simulink model "WiperMotor"  (R2025b)
settings: Solver=FixedStepDiscrete  StartTime=0.0  StopTime=20  RelTol=1e-3  EnableMultiTasking=on
settings Model: Creator=Ahmed  LastModifiedBy=Ahmed
settings DataIOCC: SaveOutput=off  SaveTime=off
settings OptimizationCC: DefaultParameterBehavior=Inlined  UseDivisionForNetSlopeComputation=on  GainParamInheritBuiltInType=on  UseFloatMulNetSlope=on  InlineInvariantSignals=on  PassReuseOutputArgsAs=Individual arguments  ZeroExternalMemoryAtStartup=off  ZeroInternalMemoryAtStartup=off  NoFixptDivByZeroProtection=on  EfficientFloat2IntCast=on  LifeSpan=1  OptimizeBlockOrder=speed  DifferentSizesBufferReuse=on  EfficientTunableParamExpr=on
settings DebuggingCC: ParameterTunabilityLossMsg=error
settings HardwareCC: ProdLongLongMode=on
settings ModelReferenceCC: ModelReferenceNumInstancesAllowed=Single
settings SFSimCC: MATLABDynamicMemAlloc=off
settings RTWCC: SystemTargetFile=ert.tlc  GenCodeOnly=on  TemplateMakefile=ert_default_tmf  GenerateReport=on  Description=Embedded Coder
settings CodeAppCC: ForceParamTrailComments=on  IgnoreCustomStorageClasses=off  OperatorAnnotations=on  SimulinkDataObjDesc=on  SFDataObjDesc=on  CustomSymbolStrGlobalVar=rt$N$M  CustomSymbolStrType=$N$M  CustomSymbolStrFcn=$N$M$F  CustomSymbolStrMacro=$N$M  InsertBlockDesc=on
settings ERTTargetCC: ERTCustomFileTemplate=example_file_process.tlc  ERTFilePackagingFormat=CompactWithDataFile  TargetLangStandard=C99 (ISO)  GenerateSampleERTMain=on  IncludeMdlTerminateFcn=off  CombineSignalStateStructs=on  SubcomponentCodeInterfacePackaging=Nonreusable function  SupportComplex=off

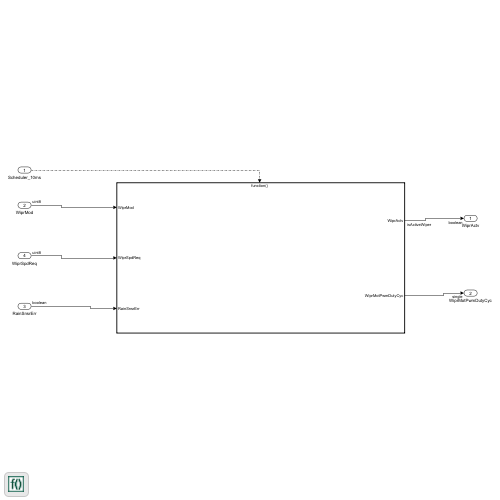
[thumbnail: Simulink's stored preview of the top-level diagram]
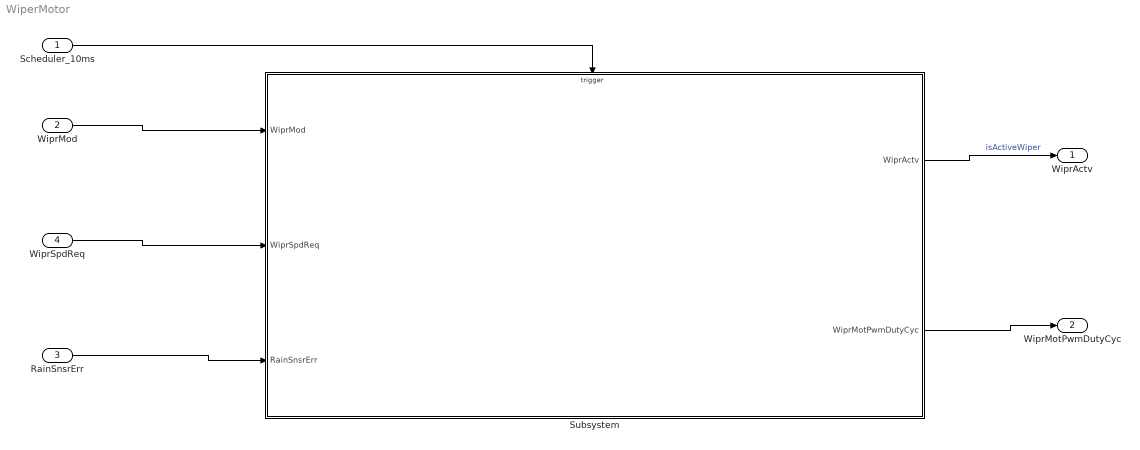
== system WiperMotor ==
  Scheduler_10ms : Inport  PortDimensions=1  OutputFunctionCall=on
  WiprMod : Inport  Port=2  OutDataTypeStr=uint8  PortDimensions=1
  RainSnsrErr : Inport  Port=3  OutDataTypeStr=boolean  PortDimensions=1
  WiprSpdReq : Inport  Port=4  OutDataTypeStr=uint8  PortDimensions=1
  Subsystem : Subsystem
  WiprActv : Outport  OutDataTypeStr=boolean  PortDimensions=1
  WiprMotPwmDutyCyc : Outport  Port=2  OutDataTypeStr=single  PortDimensions=1
  wires:
  WiprMod/1 -> Subsystem/1(WiprMod)
  WiprSpdReq/1 -> Subsystem/2(WiprSpdReq)
  RainSnsrErr/1 -> Subsystem/3(RainSnsrErr)
  Subsystem/1(WiprActv) -> WiprActv/1  "isActiveWiper"
  Subsystem/2(WiprMotPwmDutyCyc) -> WiprMotPwmDutyCyc/1
  Scheduler_10ms/1 -> Subsystem/Trigger

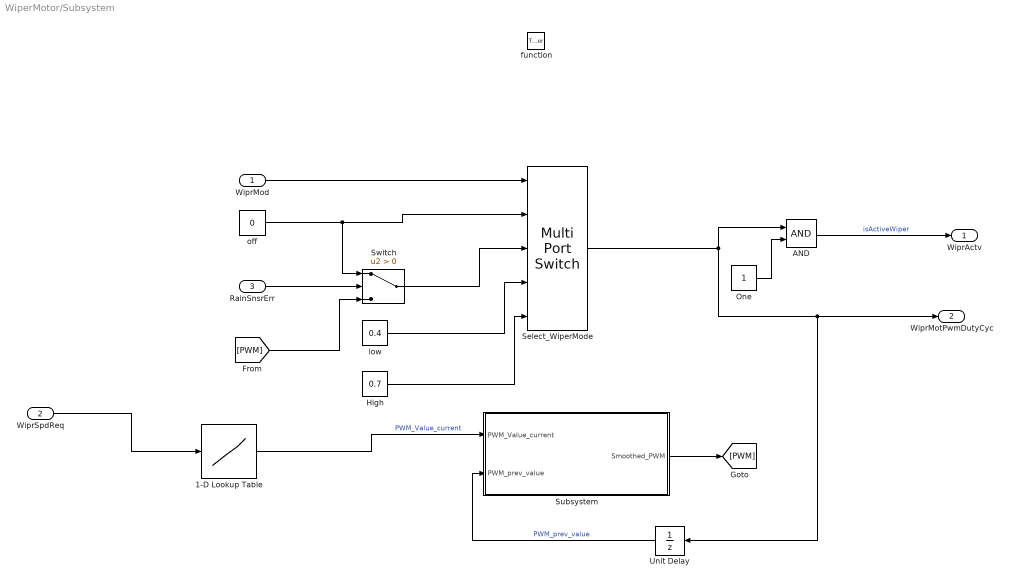
== system WiperMotor/Subsystem ==
  WiprMod : Inport
  WiprSpdReq : Inport  Port=2
  RainSnsrErr : Inport  Port=3
  function : TriggerPort  TriggerType=function-call  VariantControl=(inherit)
  1-D Lookup Table : Lookup_n-D  NumberOfTableDimensions=1  BreakpointsForDimension1=[0,1,2,3,4,5,6,7]  BreakpointsForDimension1DataTypeStr=single  Table=[0, 0.4, 0.45, 0.5, 0.55, 0.6, 0.65, 0.7]  TableDataTypeStr=single  ExtrapMethod=Clip  InternalRulePriority=Speed  OutDataTypeStr=single  RndMeth=Simplest
  AND : Logic  AllPortsSameDT=off  OutDataTypeStr=boolean
  High : Constant  Value=0.7  OutDataTypeStr=Inherit: Inherit via back propagation
  One : Constant  OutDataTypeStr=Inherit: Inherit via back propagation
  Select_WiperMode : MultiPortSwitch  DataPortOrder=Zero-based contiguous  Inputs=4  zeroidx=on  SaturateOnIntegerOverflow=off  InputSameDT=off
  Subsystem : Subsystem
  Switch : Switch  Criteria=u2 > Threshold  SaturateOnIntegerOverflow=off  InputSameDT=off
  Unit Delay : UnitDelay  SampleTime=-1  HasFrameUpgradeWarning=on
  low : Constant  Value=0.4  OutDataTypeStr=Inherit: Inherit via back propagation
  off : Constant  Value=0  OutDataTypeStr=Inherit: Inherit via back propagation
  WiprActv : Outport
  WiprMotPwmDutyCyc : Outport  Port=2
  wires:
  1-D Lookup Table/1 -> Subsystem/1(PWM_Value_current)  "PWM_Value_current"
  WiprSpdReq/1 -> 1-D Lookup Table/1
  [PWM] -> Switch/3
  Subsystem/1(Smoothed_PWM) -> [PWM]
  Unit Delay/1 -> Subsystem/2(PWM_prev_value)  "PWM_prev_value"
  AND/1 -> WiprActv/1  "isActiveWiper"
  One/1 -> AND/2
  Select_WiperMode/1 -> AND/1, WiprMotPwmDutyCyc/1, Unit Delay/1
  High/1 -> Select_WiperMode/5
  low/1 -> Select_WiperMode/4
  RainSnsrErr/1 -> Switch/2
  Switch/1 -> Select_WiperMode/3
  off/1 -> Select_WiperMode/2, Switch/1
  WiprMod/1 -> Select_WiperMode/1

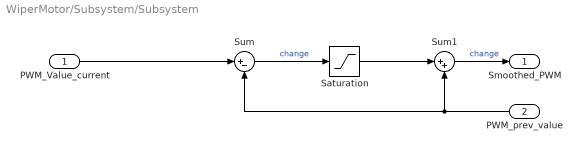
== system WiperMotor/Subsystem/Subsystem ==
  PWM_Value_current : Inport
  PWM_prev_value : Inport  Port=2
  Saturation : Saturate  UpperLimit=0.005  LowerLimit=-0.005
  Sum : Sum  Inputs=|+-
  Sum1 : Sum  Inputs=|++
  Smoothed_PWM : Outport
  wires:
  Sum1/1 -> Smoothed_PWM/1  "change"
  Saturation/1 -> Sum1/1
  PWM_Value_current/1 -> Sum/1
  PWM_prev_value/1 -> Sum1/2, Sum/2
  Sum/1 -> Saturation/1  "change"
